simulink model "implementacion_r2022a"  (R2022a)
settings: Solver=ode23t  StartTime=0.0  StopTime=inf  FixedStep=1E-4  MaxStep=100  RelTol=1e-4  EnableMultiTasking=on
InitFcn:
  | iniASU_UNIT
undefined symbols (not defined in the file or in its folder): Arrhenius, Cineticos20, Esteq, Param_ASU_D, Param_ASU_N, Param_Settler_Fns, ParamsEsteq, VarManip_D, VarManip_N, VarManip_QRF, x0_D, x0_N
libraries: dspnetwork x15
settings Model: Creator=iirizar  LastModifiedBy=goigl
settings SolverCC: InitialStep=1E-22  MaxConsecutiveMinStep=auto  AlgebraicLoopSolver=TrustRegion  SolverResetMethod=Robust
settings DataIOCC: LimitDataPoints=on  MaxDataPoints=1  SaveFinalState=on  SaveFormat=Array  SignalLoggingSaveFormat=ModelDataLogs  SaveOutput=off  SaveState=on  SignalLogging=off  SaveTime=off  ReturnWorkspaceOutputs=off
settings OptimizationCC: ExpressionDepthLimit=2147483647  LifeSpan=inf
settings DebuggingCC: UnderspecifiedInitializationDetection=Classic  MergeDetectMultiDrivingBlocksExec=none  SolverPrmCheckMsg=warning  FcnCallInpInsideContextMsg=warning  UnconnectedInputMsg=warning  UnconnectedOutputMsg=warning  UnconnectedLineMsg=warning  StateNameClashWarn=warning  SFUnexpectedBacktrackingDiag=warning  SFNoUnconditionalDefaultTransitionDiag=warning  SFExecutionAtInitializationDiag=none  SFMachineParentedDataDiag=warning  ArithmeticOperatorsInVariantConditions=warning
settings HardwareCC: ProdBitPerPointer=32  ProdBitPerSizeT=32  ProdBitPerPtrDiffT=32  ProdLargestAtomicFloat=None  ProdIntDivRoundTo=Undefined  ProdEndianess=Unspecified  ProdWordSize=32  ProdHWDeviceType=32-bit Generic
settings ModelReferenceCC: PropagateSignalLabelsOutOfModel=off
settings SFSimCC: SimUseLocalCustomCode=off  CustomCodeUndefinedFunction=UseInterfaceOnly
settings RTWCC: RTWUseLocalCustomCode=off  DLArmComputeVersion=19.05
settings CodeAppCC: StateflowObjectComments=on
settings GRTTargetCC: TargetLangStandard=C89/C90 (ANSI)  CombineOutputUpdateFcns=off  GRTInterface=on
settings ConfigComp: CovMetricSettings=dw  CovSaveCumulativeToWorkspaceVar=on  CovSaveSingleToWorkspaceVar=on  CovExternalEMLEnable=off

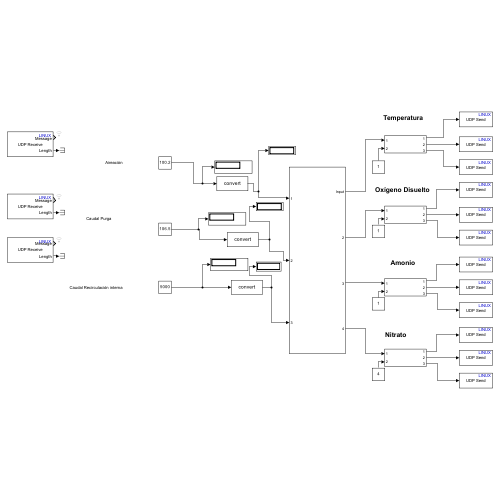
[thumbnail: Simulink's stored preview of the top-level diagram]
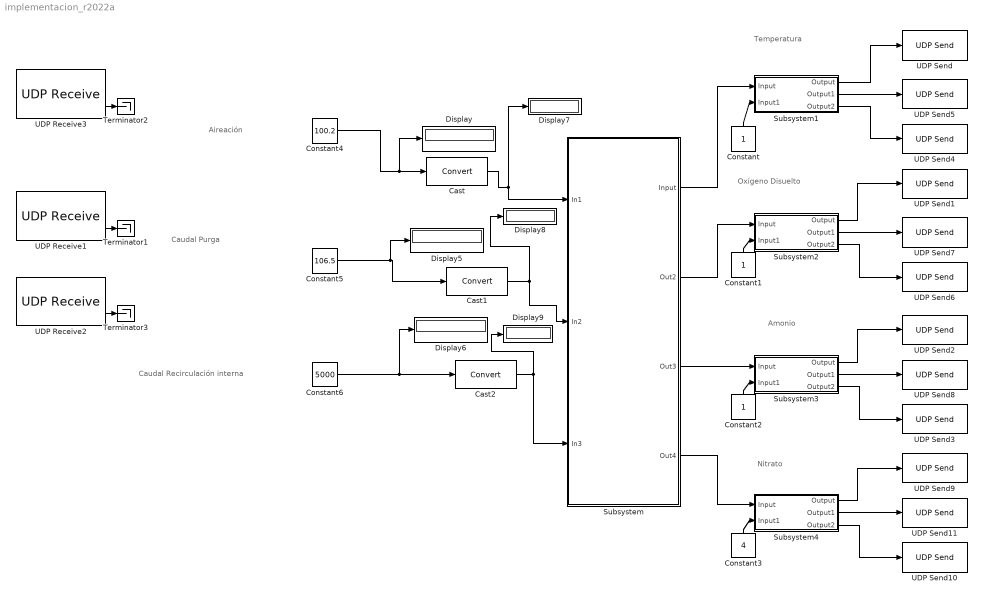
== system implementacion_r2022a ==
  note: Caudal Purga
  note: Aireación
  note: Caudal Recirculación interna
  note: Temperatura
  note: Oxígeno Disuelto
  note: Amonio
  note: Nitrato
  Cast : DataTypeConversion  OutMin=[0]  OutMax=[1000]  SaturateOnIntegerOverflow=off  RndMeth=Floor
  Cast1 : DataTypeConversion  OutMin=[0]  OutMax=[1000]  SaturateOnIntegerOverflow=off  RndMeth=Floor
  Cast2 : DataTypeConversion  OutMin=[0]  OutMax=[1000]  RndMeth=Round  SaturateOnIntegerOverflow=off
  Constant : Constant
  Constant1 : Constant
  Constant2 : Constant
  Constant3 : Constant  Value=4
  Constant4 : Constant  Value=100.2
  Constant5 : Constant  Value=106.5
  Constant6 : Constant  Value=5000
  Display{,5..9} (6 alike) : Display
  Subsystem : Subsystem
  Subsystem1 : Subsystem
  Subsystem2 : Subsystem
  Subsystem3 : Subsystem
  Subsystem4 : Subsystem
  Terminator1 : Terminator
  Terminator2 : Terminator
  Terminator3 : Terminator
  UDP Receive1 : dspnetwork/UDP Receive  localURL='0.0.0.0'  localPort=10014  remoteURL='0.0.0.0'  remotePort=-1  recvBufferSize=2  dims=1  signalDatatype=uint16  isComplex=off  isVarSize=off  showBlockingTime=on  blockingTime=0  sampletime=1  blockPlatform=LINUX
  UDP Receive2 : dspnetwork/UDP Receive  localURL='0.0.0.0'  localPort=10015  remoteURL='0.0.0.0'  remotePort=-1  recvBufferSize=2  dims=1  signalDatatype=uint16  isComplex=off  isVarSize=off  showBlockingTime=on  blockingTime=0  sampletime=1  blockPlatform=LINUX
  UDP Receive3 : dspnetwork/UDP Receive  localURL='0.0.0.0'  localPort=10013  remoteURL='0.0.0.0'  remotePort=-1  recvBufferSize=2  dims=1  signalDatatype=uint16  isComplex=off  isVarSize=off  showBlockingTime=on  blockingTime=0  sampletime=1  blockPlatform=LINUX
  UDP Send : dspnetwork/UDP Send  remoteURL='localhost'  remotePort=10001  localURL='255.255.255.255'  localPortSource=Automatically determine  localPort=-1  sendBufferSize=8192*2  sampletime=-1  blockPlatform=LINUX  separateLengthPort=0
  UDP Send1 : dspnetwork/UDP Send  remoteURL='localhost'  remotePort=10004  localURL='255.255.255.255'  localPortSource=Automatically determine  localPort=-1  sendBufferSize=8192*2  sampletime=-1  blockPlatform=LINUX  separateLengthPort=0
  UDP Send10 : dspnetwork/UDP Send  remoteURL='localhost'  remotePort=10012  localURL='255.255.255.255'  localPortSource=Automatically determine  localPort=-1  sendBufferSize=8192*2  sampletime=-1  blockPlatform=LINUX  separateLengthPort=0
  UDP Send11 : dspnetwork/UDP Send  remoteURL='localhost'  remotePort=10011  localURL='255.255.255.255'  localPortSource=Automatically determine  localPort=-1  sendBufferSize=8192*2  sampletime=-1  blockPlatform=LINUX  separateLengthPort=0
  UDP Send2 : dspnetwork/UDP Send  remoteURL='localhost'  remotePort=10007  localURL='255.255.255.255'  localPortSource=Automatically determine  localPort=-1  sendBufferSize=8192*2  sampletime=-1  blockPlatform=LINUX  separateLengthPort=0
  UDP Send3 : dspnetwork/UDP Send  remoteURL='localhost'  remotePort=10009  localURL='255.255.255.255'  localPortSource=Automatically determine  localPort=-1  sendBufferSize=8192*2  sampletime=-1  blockPlatform=LINUX  separateLengthPort=0
  UDP Send4 : dspnetwork/UDP Send  remoteURL='localhost'  remotePort=10003  localURL='255.255.255.255'  localPortSource=Automatically determine  localPort=-1  sendBufferSize=8192*2  sampletime=-1  blockPlatform=LINUX  separateLengthPort=0
  UDP Send5 : dspnetwork/UDP Send  remoteURL='localhost'  remotePort=10002  localURL='255.255.255.255'  localPortSource=Automatically determine  localPort=-1  sendBufferSize=8192*2  sampletime=-1  blockPlatform=LINUX  separateLengthPort=0
  UDP Send6 : dspnetwork/UDP Send  remoteURL='localhost'  remotePort=10006  localURL='255.255.255.255'  localPortSource=Automatically determine  localPort=-1  sendBufferSize=8192*2  sampletime=-1  blockPlatform=LINUX  separateLengthPort=0
  UDP Send7 : dspnetwork/UDP Send  remoteURL='localhost'  remotePort=10005  localURL='255.255.255.255'  localPortSource=Automatically determine  localPort=-1  sendBufferSize=8192*2  sampletime=-1  blockPlatform=LINUX  separateLengthPort=0
  UDP Send8 : dspnetwork/UDP Send  remoteURL='localhost'  remotePort=10008  localURL='255.255.255.255'  localPortSource=Automatically determine  localPort=-1  sendBufferSize=8192*2  sampletime=-1  blockPlatform=LINUX  separateLengthPort=0
  UDP Send9 : dspnetwork/UDP Send  remoteURL='localhost'  remotePort=10010  localURL='255.255.255.255'  localPortSource=Automatically determine  localPort=-1  sendBufferSize=8192*2  sampletime=-1  blockPlatform=LINUX  separateLengthPort=0
  wires:
  UDP Receive1/2 -> Terminator1/1
  UDP Receive2/2 -> Terminator3/1
  Cast/1 -> Display7/1, Subsystem/1(In1)
  Cast1/1 -> Display8/1, Subsystem/2(In2)
  Cast2/1 -> Display9/1, Subsystem/3(In3)
  Subsystem/1(Input) -> Subsystem1/1(Input)
  Subsystem1/1(Output) -> UDP Send/1
  Subsystem1/2(Output1) -> UDP Send5/1
  Subsystem1/3(Output2) -> UDP Send4/1
  Constant/1 -> Subsystem1/2(Input1)
  Constant1/1 -> Subsystem2/2(Input1)
  Subsystem2/1(Output) -> UDP Send1/1
  Subsystem2/2(Output1) -> UDP Send7/1
  Subsystem2/3(Output2) -> UDP Send6/1
  Subsystem/2(Out2) -> Subsystem2/1(Input)
  Subsystem3/2(Output1) -> UDP Send8/1
  Subsystem3/3(Output2) -> UDP Send3/1
  Subsystem3/1(Output) -> UDP Send2/1
  Subsystem/3(Out3) -> Subsystem3/1(Input)
  Constant2/1 -> Subsystem3/2(Input1)
  Subsystem4/2(Output1) -> UDP Send11/1
  Subsystem4/3(Output2) -> UDP Send10/1
  Subsystem4/1(Output) -> UDP Send9/1
  Subsystem/4(Out4) -> Subsystem4/1(Input)
  Constant3/1 -> Subsystem4/2(Input1)
  UDP Receive3/2 -> Terminator2/1
  Constant4/1 -> Display/1, Cast/1
  Constant5/1 -> Display5/1, Cast1/1
  Constant6/1 -> Display6/1, Cast2/1

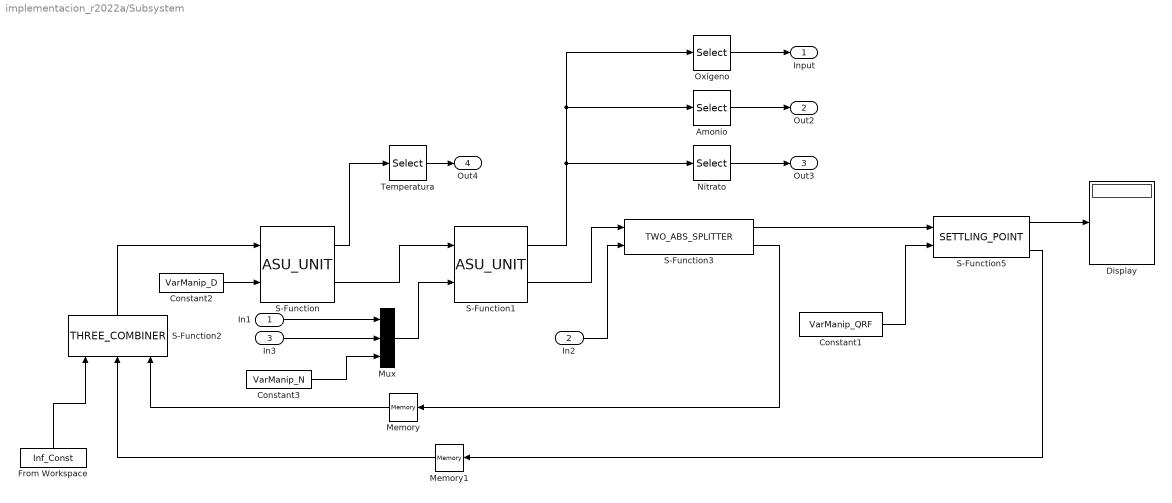
== system implementacion_r2022a/Subsystem ==
  In1 : Inport
  In2 : Inport  Port=2
  In3 : Inport  Port=3
  Amonio : Selector  InputPortWidth=9  IndexOptions=Index vector (dialog)  Indices=[4]  OutputSizes=1
  Constant1 : Constant  Value=VarManip_QRF
  Constant2 : Constant  Value=VarManip_D
  Constant3 : Constant  Value=VarManip_N
  Display : Display
  From Workspace : FromWorkspace  VariableName=Inf_Const  Interpolate=off  OutputAfterFinalValue=Holding final value
  Memory : Memory  InheritSampleTime=on
  Memory1 : Memory  InheritSampleTime=on
  Mux : Mux  Inputs=3
  Nitrato : Selector  InputPortWidth=9  IndexOptions=Index vector (dialog)  Indices=[3]  OutputSizes=1
  Oxígeno : Selector  InputPortWidth=9  IndexOptions=Index vector (dialog)  Indices=[5]  OutputSizes=1
  S-Function : S-Function  FunctionName=ASU_UNIT  Parameters=ParamsEsteq,Cineticos20,Arrhenius,Esteq,Param_ASU_D,x0_D  SFunctionDeploymentMode=off  EnableBusSupport=off
  S-Function1 : S-Function  FunctionName=ASU_UNIT  Parameters=ParamsEsteq,Cineticos20,Arrhenius,Esteq,Param_ASU_N,x0_N  SFunctionDeploymentMode=off  EnableBusSupport=off
  S-Function2 : S-Function  FunctionName=THREE_COMBINER  SFunctionDeploymentMode=off  EnableBusSupport=off
  S-Function3 : S-Function  FunctionName=TWO_ABS_SPLITTER  SFunctionDeploymentMode=off  EnableBusSupport=off
  S-Function5 : S-Function  FunctionName=SETTLING_POINT  Parameters=ParamsEsteq,Param_Settler_Fns  SFunctionDeploymentMode=off  EnableBusSupport=off
  Temperatura : Selector  InputPortWidth=9  IndexOptions=Index vector (dialog)  Indices=[8]  OutputSizes=1
  Input : Outport
  Out2 : Outport  Port=2
  Out3 : Outport  Port=3
  Out4 : Outport  Port=4
  wires:
  Constant2/1 -> S-Function/2
  Constant1/1 -> S-Function5/2
  In1/1 -> Mux/1
  Mux/1 -> S-Function1/2
  Constant3/1 -> Mux/3
  S-Function/2 -> S-Function1/1
  S-Function5/1 -> Display/1
  Memory1/1 -> S-Function2/2
  S-Function2/1 -> S-Function/1
  Memory/1 -> S-Function2/3
  S-Function5/3 -> Memory1/1
  S-Function1/2 -> S-Function3/1
  S-Function3/2 -> Memory/1
  S-Function3/1 -> S-Function5/1
  From Workspace/1 -> S-Function2/1
  In2/1 -> S-Function3/2
  In3/1 -> Mux/2
  S-Function1/1 -> Nitrato/1, Amonio/1, Oxígeno/1
  S-Function/1 -> Temperatura/1
  Nitrato/1 -> Out3/1
  Amonio/1 -> Out2/1
  Oxígeno/1 -> Input/1
  Temperatura/1 -> Out4/1

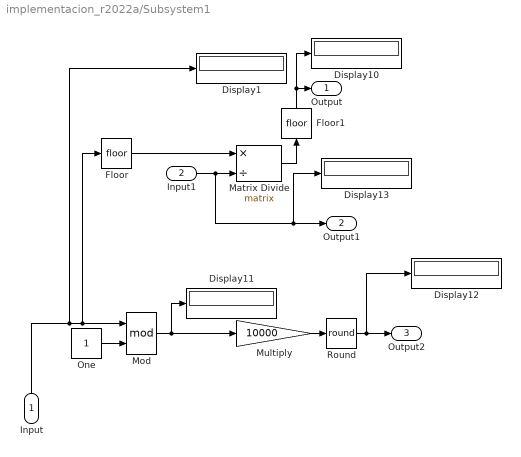
== system implementacion_r2022a/Subsystem1 ==
  Input : Inport
  Input1 : Inport  Port=2
  Display{1,10..13} (5 alike) : Display
  Floor : Rounding
  Floor1 : Rounding
  Matrix Divide : Product  Inputs=*/  Multiplication=Matrix(*)
  Mod : Math  Operator=mod
  Multiply : Gain  Gain=10000
  One : Constant  OutDataTypeStr=Inherit: Inherit via back propagation
  Round : Rounding  Operator=round
  Output : Outport
  Output1 : Outport  Port=2
  Output2 : Outport  Port=3
  wires:
  Floor/1 -> Matrix Divide/1
  Input1/1 -> Matrix Divide/2, Output1/1, Display13/1
  Multiply/1 -> Round/1
  Round/1 -> Output2/1, Display12/1
  Input/1 -> Display1/1, Floor/1, Mod/1
  One/1 -> Mod/2
  Mod/1 -> Multiply/1, Display11/1
  Matrix Divide/1 -> Floor1/1
  Floor1/1 -> Output/1, Display10/1

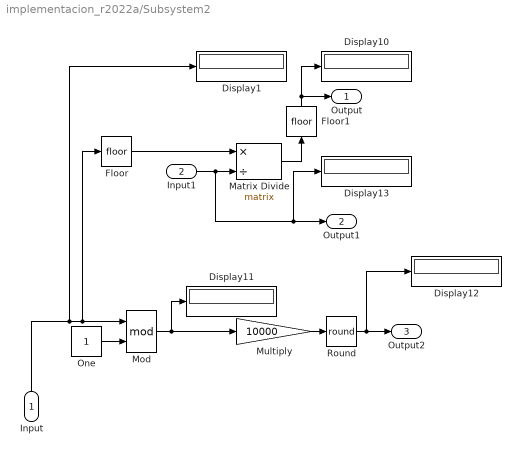
== system implementacion_r2022a/Subsystem2 ==
  Input : Inport
  Input1 : Inport  Port=2
  Display{1,10..13} (5 alike) : Display
  Floor : Rounding
  Floor1 : Rounding
  Matrix Divide : Product  Inputs=*/  Multiplication=Matrix(*)
  Mod : Math  Operator=mod
  Multiply : Gain  Gain=10000
  One : Constant  OutDataTypeStr=Inherit: Inherit via back propagation
  Round : Rounding  Operator=round
  Output : Outport
  Output1 : Outport  Port=2
  Output2 : Outport  Port=3
  wires:
  Floor/1 -> Matrix Divide/1
  Input1/1 -> Matrix Divide/2, Output1/1, Display13/1
  Multiply/1 -> Round/1
  Round/1 -> Output2/1, Display12/1
  Input/1 -> Display1/1, Floor/1, Mod/1
  One/1 -> Mod/2
  Mod/1 -> Multiply/1, Display11/1
  Matrix Divide/1 -> Floor1/1
  Floor1/1 -> Display10/1, Output/1

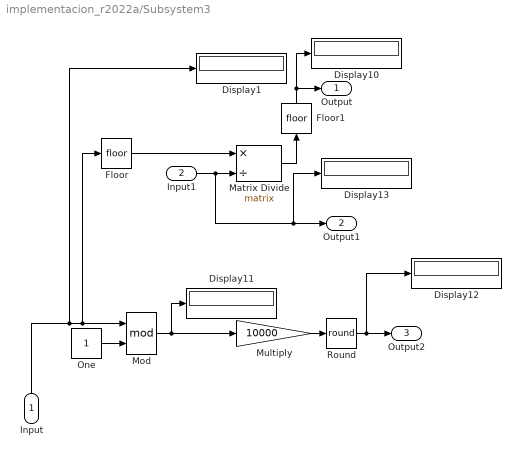
== system implementacion_r2022a/Subsystem3 ==
  Input : Inport
  Input1 : Inport  Port=2
  Display{1,10..13} (5 alike) : Display
  Floor : Rounding
  Floor1 : Rounding
  Matrix Divide : Product  Inputs=*/  Multiplication=Matrix(*)
  Mod : Math  Operator=mod
  Multiply : Gain  Gain=10000
  One : Constant  OutDataTypeStr=Inherit: Inherit via back propagation
  Round : Rounding  Operator=round
  Output : Outport
  Output1 : Outport  Port=2
  Output2 : Outport  Port=3
  wires:
  Floor/1 -> Matrix Divide/1
  Input1/1 -> Matrix Divide/2, Output1/1, Display13/1
  Multiply/1 -> Round/1
  Round/1 -> Output2/1, Display12/1
  Input/1 -> Display1/1, Floor/1, Mod/1
  One/1 -> Mod/2
  Mod/1 -> Multiply/1, Display11/1
  Matrix Divide/1 -> Floor1/1
  Floor1/1 -> Output/1, Display10/1

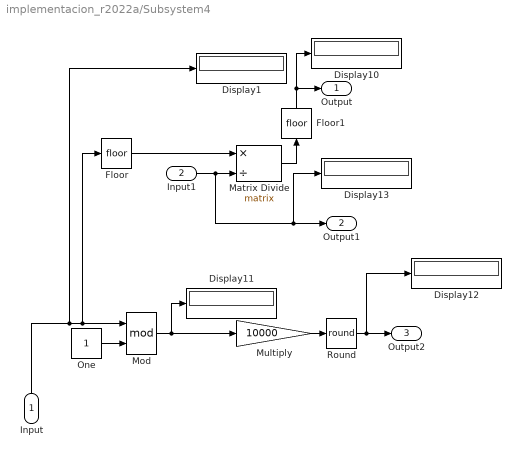
== system implementacion_r2022a/Subsystem4 ==
  Input : Inport
  Input1 : Inport  Port=2
  Display{1,10..13} (5 alike) : Display
  Floor : Rounding
  Floor1 : Rounding
  Matrix Divide : Product  Inputs=*/  Multiplication=Matrix(*)
  Mod : Math  Operator=mod
  Multiply : Gain  Gain=10000
  One : Constant  OutDataTypeStr=Inherit: Inherit via back propagation
  Round : Rounding  Operator=round
  Output : Outport
  Output1 : Outport  Port=2
  Output2 : Outport  Port=3
  wires:
  Floor/1 -> Matrix Divide/1
  Input1/1 -> Matrix Divide/2, Output1/1, Display13/1
  Multiply/1 -> Round/1
  Round/1 -> Output2/1, Display12/1
  Input/1 -> Display1/1, Floor/1, Mod/1
  One/1 -> Mod/2
  Mod/1 -> Multiply/1, Display11/1
  Matrix Divide/1 -> Floor1/1
  Floor1/1 -> Output/1, Display10/1
